simulink model "hw2_simulink"  (R2021b)
settings: Solver=VariableStepAuto  StartTime=0.0  StopTime=500  RelTol=1e-3
settings Model: PacingRate=100  Creator=admin  LastModifiedBy=Parsa_The_Conqeuror

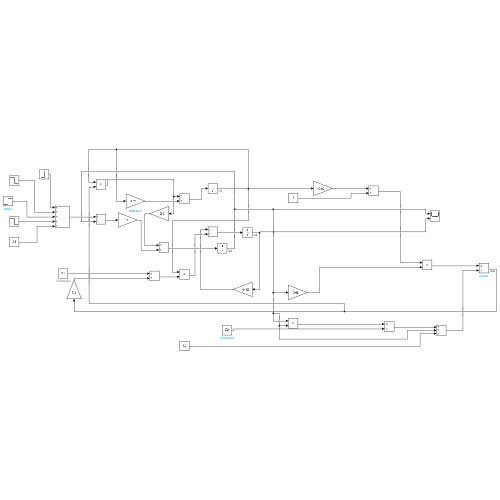
[thumbnail: Simulink's stored preview of the top-level diagram]
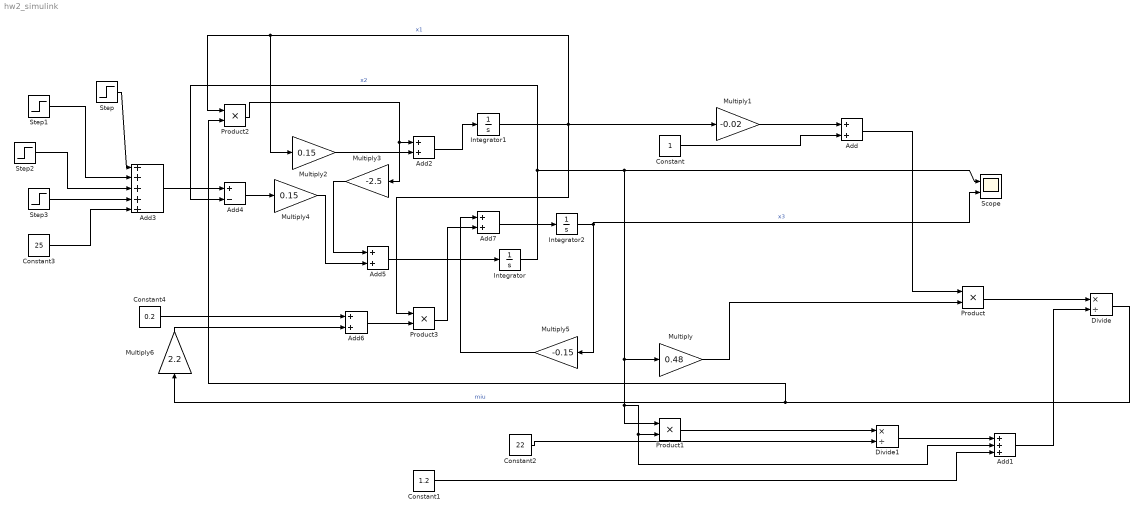
== system hw2_simulink ==
  Add{,2,5..7} (5 alike) : Sum
  Add1 : Sum  Inputs=+++
  Add3 : Sum  Inputs=+++++
  Add4 : Sum  Inputs=+-
  Constant : Constant
  Constant1 : Constant  Value=1.2
  Constant2 : Constant  Value=22
  Constant3 : Constant  Value=25
  Constant4 : Constant  Value=0.2
  Divide : Product  Inputs=*/
  Divide1 : Product  Inputs=*/
  Integrator : Integrator
  Integrator1 : Integrator
  Integrator2 : Integrator
  Multiply : Gain  Gain=0.48
  Multiply1 : Gain  Gain=-0.02
  Multiply2 : Gain  Gain=0.15
  Multiply3 : Gain  Gain=-2.5
  Multiply4 : Gain  Gain=0.15
  Multiply5 : Gain  Gain=-0.15
  Multiply6 : Gain  Gain=2.2
  Product{,1..3} (4 alike) : Product
  Scope : Scope  NumInputPorts=2
  Step : Step  Time=100  After=5  SampleTime=0
  Step1 : Step  Time=200  After=-5  SampleTime=0
  Step2 : Step  Time=400  After=5  SampleTime=0
  Step3 : Step  Time=300  After=-5  SampleTime=0
  wires:
  Integrator/1 -> Add4/2, Scope/1, Product1/1, Product1/2, Add1/2, Multiply/1  "x2"
  Integrator1/1 -> Product3/1, Multiply2/1, Product2/1, Multiply1/1  "x1"
  Integrator2/1 -> Multiply5/1, Scope/2  "x3"
  Multiply/1 -> Product/2
  Add/1 -> Product/1
  Constant/1 -> Add/2
  Multiply1/1 -> Add/1
  Product/1 -> Divide/1
  Constant1/1 -> Add1/3
  Product1/1 -> Divide1/1
  Divide1/1 -> Add1/1
  Constant2/1 -> Divide1/2
  Divide/1 -> Product2/2, Multiply6/1  "miu"
  Add1/1 -> Divide/2
  Product2/1 -> Multiply3/1, Add2/1
  Add2/1 -> Integrator1/1
  Step/1 -> Add3/1
  Step1/1 -> Add3/2
  Step2/1 -> Add3/3
  Step3/1 -> Add3/4
  Constant3/1 -> Add3/5
  Multiply2/1 -> Add2/2
  Multiply3/1 -> Add5/1
  Add3/1 -> Add4/1
  Add4/1 -> Multiply4/1
  Add5/1 -> Integrator/1
  Multiply4/1 -> Add5/2
  Multiply5/1 -> Add7/1
  Constant4/1 -> Add6/1
  Multiply6/1 -> Add6/2
  Add6/1 -> Product3/2
  Product3/1 -> Add7/2
  Add7/1 -> Integrator2/1
